simulink model "Template_v3_03_2020a"  (R2020a)
settings: Solver=ode4  StartTime=0.0  StopTime=tsim  FixedStep=baseRate  RelTol=1e-3  EnableMultiTasking=on
values from neighbouring files (symbols this model uses):
  baseRate = 0.05    [Run_Initializer.m]
  dockDist = 0.5    [Run_Initializer.m]
  drop_states_BLACK = [ 1.19; 1.45; -0.06737]    [Run_Initializer.m]
  drop_states_BLUE = [ 0.52; 1.45; -0.06737]    [Run_Initializer.m]
  drop_states_RED = [ 2.114; 1.46; -3.113]    [Run_Initializer.m]
  F_thrusters_BLACK = 0.25.*ones(8,1)    [Run_Initializer.m]
  F_thrusters_BLUE = 0.25.*ones(8,1)    [Run_Initializer.m]
  F_thrusters_RED = 0.25.*ones(8,1)    [Run_Initializer.m]
  final_states_BLACK = [1; 0.5; (0/180*pi)]    [Run_Initializer.m]
  fixed_att = init_states_RED(3)    [Run_Initializer.m]
  guess = [8.968203153403679e+02,-2.543974115068790e+03,0.235869606391541,0.474952865321742,0.474987768379695,0.520000000000000,0.485664087948638,0,0,.1,.1,.1,.1,.1,.1,.1,.1,.1,.1,.1,.1,.1,.1,.1,.1,.1,.2]    [Run_Initializer.m]
  home_states_BLACK = [ xLength/2; yLength/2; 0]    [Run_Initializer.m]
  home_states_BLUE = [ xLength/2-0.4; yLength/2; 0]    [Run_Initializer.m]
  home_states_RED = [ xLength/2+0.4; yLength/2; pi]    [Run_Initializer.m]
  init_states_BLACK = [0.5; 0.5; (0/180*pi)]    [Run_Initializer.m]
  init_states_BLUE = [ xLength/2-0.7; yLength/2; 0]    [Run_Initializer.m]
  init_states_RED = [ 3; 2; 0]    [Run_Initializer.m]
  Kd_tb = 0.4    [Run_Initializer.m]
  Kd_tblue = 0.4    [Run_Initializer.m]
  Kd_tr = 0.4    [Run_Initializer.m]
  Kd_xb = 5    [Run_Initializer.m]
  Kd_xblue = 5    [Run_Initializer.m]
  Kd_xr = 5    [Run_Initializer.m]
  Kd_yb = 5    [Run_Initializer.m]
  Kd_yblue = 5    [Run_Initializer.m]
  Kd_yr = 5    [Run_Initializer.m]
  Kp_tb = 0.1    [Run_Initializer.m]
  Kp_tblue = 0.1    [Run_Initializer.m]
  Kp_tr = 0.1    [Run_Initializer.m]
  Kp_xb = 2    [Run_Initializer.m]
  Kp_xblue = 2    [Run_Initializer.m]
  Kp_xr = 2    [Run_Initializer.m]
  Kp_yb = 2    [Run_Initializer.m]
  Kp_yblue = 2    [Run_Initializer.m]
  Kp_yr = 2    [Run_Initializer.m]
  max_force = F_thrusters_RED(1)*2 * 0.95    [Run_Initializer.m]
  max_torque = 0.13*4    (= 0.52)    [Run_Initializer.m]
  moving_BLACK = [(final_states_BLACK(1)-init_states_BLACK(1))/Phase3_SubPhase2_Duration,(final_states_BLACK(2)-init_states_BLACK(2))/Phase3_SubPhase2_Duration,0]    [Run_Initializer.m]
  noise_variance_BLACK = 0    [Run_Initializer.m]
  noise_variance_BLUE = 0    [Run_Initializer.m]
  noise_variance_RED = 0    [Run_Initializer.m]
  Phase0_End = Phase0_Duration    (= 10)    [Run_Initializer.m]
  Phase1_End = Phase0_Duration + Phase1_Duration    (= 15)    [Run_Initializer.m]
  Phase2_End = Phase0_Duration + Phase1_Duration +                                   Phase2_Duration    (= 35)    [Run_Initializer.m]
  Phase3_Duration = 85    [Run_Initializer.m]
  Phase3_End = Phase0_Duration + Phase1_Duration +                                   Phase2_Duration + Phase3_Duration    (= 120)    [Run_Initializer.m]
  Phase3_SubPhase1_End = Phase2_End + Phase3_SubPhase1_Duration    (= 40)    [Run_Initializer.m]
  Phase3_SubPhase2_Duration = 70    [Run_Initializer.m]
  Phase3_SubPhase2_End = Phase2_End + Phase3_SubPhase1_Duration +                                   Phase3_SubPhase2_Duration    (= 110)    [Run_Initializer.m]
  Phase3_SubPhase3_End = Phase2_End + Phase3_SubPhase1_Duration +                                   Phase3_SubPhase2_Duration +                                  Phase3_SubPhase3_Duration    (= 120)    [Run_Initializer.m]
  Phase3_SubPhase4_End = Phase2_End + Phase3_SubPhase1_Duration +                                   Phase3_SubPhase2_Duration +                                  Phase3_SubPhase3_Duration +                                  Phase3_SubPhase4_Duration    [Run_Initializer.m]
  Phase4_End = Phase0_Duration + Phase1_Duration +                                   Phase2_Duration + Phase3_Duration +                                   Phase4_Duration    (= 140)    [Run_Initializer.m]
  Phase5_End = Phase0_Duration + Phase1_Duration +                                   Phase2_Duration + Phase3_Duration +                                   Phase4_Duration + Phase5_Duration    (= 145)    [Run_Initializer.m]
  REDInertia = 0.2709    [Run_Initializer.m]
  REDMass = 16.9478    [Run_Initializer.m]
  serverRate = 0.1    [Run_Initializer.m]
  thruster_dist2CG_BLACK = [83.42;-52.58;55.94;-60.05;54.08;-53.92;77.06;-55.94]    [Run_Initializer.m]
  thruster_dist2CG_BLUE = [83.42;-52.58;55.94;-60.05;54.08;-53.92;77.06;-55.94]    [Run_Initializer.m]
  thruster_dist2CG_RED = [49.92;-78.08;70.46;-63.54;81.08;-50.42;57.44;-75.96]    [Run_Initializer.m]
  tolSGRA = [Er; Eg]    [Run_Initializer.m]
  xLength = 3.51155    [Run_Initializer.m]
  yLength = 2.41935    [Run_Initializer.m]
undefined symbols (not defined in the file or in its folder): DiscIntNeverNeededParam, platformSelection, simMode, WhoAmI
libraries: embdlinuxlib x11, raspberrypiBasiclib x10, dspsigops x3, dspswit3 x2, MainLibrary x2, simulink x1
(part 2 of 9)

== system Template_v3_03_2020a/Real-Time Visualization ==
  Set Universal Time (If this is a simulation) : Clock
  UDP Send : embdlinuxlib/UDP Send  remoteURL='172.24.1.102'  remotePort=26000  localURL='0.0.0.0'  localPortSource=Automatically determine  localPort=-1  sampletime=-1  blockPlatform=Raspberry Pi  separateLengthPort=0
      settings: SourceProductBaseCode=SC_BEAGLEBONE_BLUE,RASPPI
  wires:
  Set Universal Time (If this is a simulation)/1 -> UDP Send/1

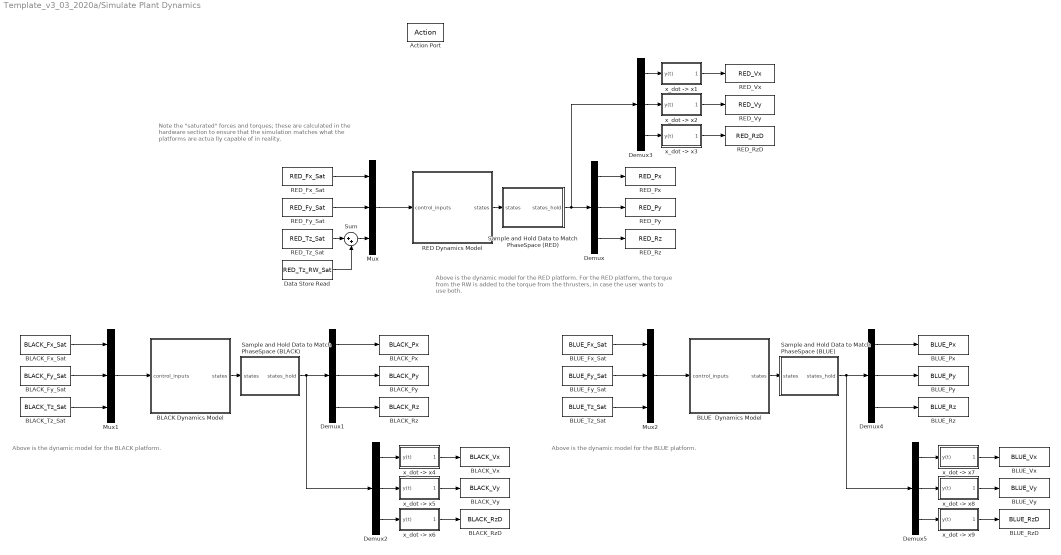
== system Template_v3_03_2020a/Simulate Plant Dynamics ==
  note: Above is the dynamic model for the RED
      | platform. For the RED platform, the torque from the RW is added to the torque from the thrusters, in case the user wants to use both.
  note: Above is the dynamic model for the BLACK platform.
  note: Note the "saturated" forces and torques; these are calculated in the hardware section to ensure that the simulation matches what the platforms are actua lly capable of in reality.
  note: Above is the dynamic model for the BLUE platform.
  Action Port : ActionPort  ActionPortLabel=if(u1 == 1)
  BLACK Dynamics Model : Subsystem  SystemSampleTime=serverRate
  BLACK_Fx_Sat : DataStoreRead  DataStoreName=BLACK_Fx_Sat
  BLACK_Fy_Sat : DataStoreRead  DataStoreName=BLACK_Fy_Sat
  BLACK_Px : DataStoreWrite  DataStoreName=BLACK_Px
  BLACK_Py : DataStoreWrite  DataStoreName=BLACK_Py
  BLACK_Rz : DataStoreWrite  DataStoreName=BLACK_Rz
  BLACK_RzD : DataStoreWrite  DataStoreName=BLACK_RzD
  BLACK_Tz_Sat : DataStoreRead  DataStoreName=BLACK_Tz_Sat
  BLACK_Vx : DataStoreWrite  DataStoreName=BLACK_Vx
  BLACK_Vy : DataStoreWrite  DataStoreName=BLACK_Vy
  BLUE  Dynamics Model : Subsystem  SystemSampleTime=serverRate
  "BLUE_Fx_Sat " : DataStoreRead  DataStoreName=BLUE_Fx_Sat
  BLUE_Fy_Sat : DataStoreRead  DataStoreName=BLUE_Fy_Sat
  "BLUE_Px " : DataStoreWrite  DataStoreName=BLUE_Px
  BLUE_Py : DataStoreWrite  DataStoreName=BLUE_Py
  BLUE_Rz : DataStoreWrite  DataStoreName=BLUE_Rz
  BLUE_RzD : DataStoreWrite  DataStoreName=BLUE_RzD
  BLUE_Tz_Sat : DataStoreRead  DataStoreName=BLUE_Tz_Sat
  BLUE_Vx : DataStoreWrite  DataStoreName=BLUE_Vx
  BLUE_Vy : DataStoreWrite  DataStoreName=BLUE_Vy
  Data Store Read : DataStoreRead  DataStoreName=RED_Tz_RW_Sat
  Demux{,1..5} (6 alike) : Demux  Outputs=3
  Mux : Mux  Inputs=3
  Mux1 : Mux  Inputs=3
  Mux2 : Mux  Inputs=3
  RED Dynamics Model : Subsystem  SystemSampleTime=serverRate
  RED_Fx_Sat : DataStoreRead  DataStoreName=RED_Fx_Sat
  RED_Fy_Sat : DataStoreRead  DataStoreName=RED_Fy_Sat
  RED_Px : DataStoreWrite  DataStoreName=RED_Px
  RED_Py : DataStoreWrite  DataStoreName=RED_Py
  RED_Rz : DataStoreWrite  DataStoreName=RED_Rz
  RED_RzD : DataStoreWrite  DataStoreName=RED_RzD
  RED_Tz_Sat : DataStoreRead  DataStoreName=RED_Tz_Sat
  RED_Vx : DataStoreWrite  DataStoreName=RED_Vx
  RED_Vy : DataStoreWrite  DataStoreName=RED_Vy
  Sample and Hold Data to Match PhaseSpace (BLACK) : Subsystem
  Sample and Hold Data to Match PhaseSpace (BLUE) : Subsystem
  Sample and Hold Data to Match PhaseSpace (RED) : Subsystem
  Sum : Sum  Inputs=|++
  "x_dot -> x1" : Subsystem
  "x_dot -> x2" : Subsystem
  "x_dot -> x3" : Subsystem
  "x_dot -> x4" : Subsystem
  "x_dot -> x5" : Subsystem
  "x_dot -> x6" : Subsystem
  "x_dot -> x7" : Subsystem
  "x_dot -> x8" : Subsystem
  "x_dot -> x9" : Subsystem
  wires:
  Demux/3 -> RED_Rz/1
  RED_Fx_Sat/1 -> Mux/1
  BLACK_Fy_Sat/1 -> Mux1/2
  BLACK_Tz_Sat/1 -> Mux1/3
  RED_Fy_Sat/1 -> Mux/2
  BLACK_Fx_Sat/1 -> Mux1/1
  Demux/2 -> RED_Py/1
  Demux/1 -> RED_Px/1
  Demux1/1 -> BLACK_Px/1
  Demux1/2 -> BLACK_Py/1
  Demux1/3 -> BLACK_Rz/1
  RED_Tz_Sat/1 -> Sum/1
  Sum/1 -> Mux/3
  Data Store Read/1 -> Sum/2
  Demux2/1 -> "x_dot -> x4"/1(y(t))
  Demux2/2 -> "x_dot -> x5"/1(y(t))
  Demux2/3 -> "x_dot -> x6"/1(y(t))
  Demux3/2 -> "x_dot -> x2"/1(y(t))
  Demux3/1 -> "x_dot -> x1"/1(y(t))
  Demux3/3 -> "x_dot -> x3"/1(y(t))
  "x_dot -> x1"/1(dy(t)/dt) -> RED_Vx/1
  "x_dot -> x2"/1(dy(t)/dt) -> RED_Vy/1
  "x_dot -> x3"/1(dy(t)/dt) -> RED_RzD/1
  "x_dot -> x4"/1(dy(t)/dt) -> BLACK_Vx/1
  "x_dot -> x5"/1(dy(t)/dt) -> BLACK_Vy/1
  "x_dot -> x6"/1(dy(t)/dt) -> BLACK_RzD/1
  Mux/1 -> RED Dynamics Model/1(control_inputs)
  Mux1/1 -> BLACK Dynamics Model/1(control_inputs)
  Sample and Hold Data to Match PhaseSpace (BLACK)/1(states_hold) -> Demux2/1, Demux1/1
  BLACK Dynamics Model/1(states) -> Sample and Hold Data to Match PhaseSpace (BLACK)/1(states)
  Sample and Hold Data to Match PhaseSpace (RED)/1("states_hold ") -> Demux3/1, Demux/1
  RED Dynamics Model/1(states) -> Sample and Hold Data to Match PhaseSpace (RED)/1(states)
  Demux4/3 -> BLUE_Rz/1
  Demux5/3 -> "x_dot -> x9"/1(y(t))
  Demux4/1 -> "BLUE_Px "/1
  "x_dot -> x9"/1(dy(t)/dt) -> BLUE_RzD/1
  "x_dot -> x8"/1(dy(t)/dt) -> BLUE_Vy/1
  BLUE  Dynamics Model/1(states) -> Sample and Hold Data to Match PhaseSpace (BLUE)/1(states)
  Sample and Hold Data to Match PhaseSpace (BLUE)/1(states_hold) -> Demux5/1, Demux4/1
  "BLUE_Fx_Sat "/1 -> Mux2/1
  BLUE_Fy_Sat/1 -> Mux2/2
  BLUE_Tz_Sat/1 -> Mux2/3
  Mux2/1 -> BLUE  Dynamics Model/1(control_inputs)
  Demux5/1 -> "x_dot -> x7"/1(y(t))
  Demux5/2 -> "x_dot -> x8"/1(y(t))
  "x_dot -> x7"/1(dy(t)/dt) -> BLUE_Vx/1
  Demux4/2 -> BLUE_Py/1

== system Template_v3_03_2020a/Subsystem ==
  Universal_Time : DataStoreRead  DataStoreName=Univ_Time
  Time : Outport  VectorParamsAs1DForOutWhenUnconnected=off
  wires:
  Universal_Time/1 -> Time/1

== system Template_v3_03_2020a/Float & Magnet Controls/Change RED Behavior ==
  Action Port : ActionPort  ActionPortLabel=if(u1 == 0)
  Data Store Read : DataStoreRead  DataStoreName=Magnet_State
  Data Store Read1 : DataStoreRead  DataStoreName=Float_State
  GPIO for Magnet : embdlinuxlib/GPIO Write  board=Pi 3 Model B  gpio=10  direction=Output  blockPlatform=Raspberry Pi
      settings: SourceProductBaseCode=SC_BEAGLEBONE_BLUE,RASPPI
  GPIO for Pucks : embdlinuxlib/GPIO Write  board=Pi 3 Model B  gpio=26  direction=Output  blockPlatform=Raspberry Pi
      settings: SourceProductBaseCode=SC_BEAGLEBONE_BLUE,RASPPI
  wires:
  Data Store Read1/1 -> GPIO for Pucks/1
  Data Store Read/1 -> GPIO for Magnet/1

== system Template_v3_03_2020a/Float & Magnet Controls/Is this a simulation? ==
  Constant : Constant  Value=simMode  SampleTime=-1
  isSim : Outport  VectorParamsAs1DForOutWhenUnconnected=off
  wires:
  Constant/1 -> isSim/1

== system Template_v3_03_2020a/From Force//Torque to PWM Signal/Change BLACK Behavior ==
  note: Calculate the percentage of time each thruster must be on, and send to the PWM blocks.
  note: Using the attitude, rotate the forces into the body frame.
  note: Calculate which thrusters must be turned on and for how long.
  Action Port : ActionPort  ActionPortLabel=if(u1 == 2 | u2 == 1)
  BLACK_Fx : DataStoreRead  DataStoreName=BLACK_Fx
  BLACK_Fy : DataStoreRead  DataStoreName=BLACK_Fy
  BLACK_Rz : DataStoreRead  DataStoreName=BLACK_Rz
  BLACK_Tz : DataStoreRead  DataStoreName=BLACK_Tz
  Calculate Thruster ON/OFF : Subsystem
  Mux : Mux  Inputs=2
  Mux1 : Mux  Inputs=2
  Rotate Forces to Body : Subsystem
  BLACK PWM : Outport  VectorParamsAs1DForOutWhenUnconnected=off
  wires:
  Rotate Forces to Body/1(F_b) -> Mux1/1
  BLACK_Fx/1 -> Mux/1
  Calculate Thruster ON/OFF/1(ThrusterPWM) -> BLACK PWM/1
  BLACK_Rz/1 -> Rotate Forces to Body/2(Rz)
  Mux/1 -> Rotate Forces to Body/1("F_I ")
  BLACK_Tz/1 -> Mux1/2
  Mux1/1 -> Calculate Thruster ON/OFF/1("[Fx_b; Fy_b; Tz]")
  BLACK_Fy/1 -> Mux/2

== system Template_v3_03_2020a/From Force//Torque to PWM Signal/Change BLUE Behavior ==
  note: Calculate the percentage of time each thruster must be on, and send to the PWM blocks.
  note: Using the attitude, rotate the forces into the body frame.
  note: Calculate which thrusters must be turned on and for how long.
  Action Port : ActionPort  ActionPortLabel=if(u1 == 3 | u2 == 1)
  BLUE_Fx : DataStoreRead  DataStoreName=BLUE_Fx
  BLUE_Fy : DataStoreRead  DataStoreName=BLUE_Fy
  BLUE_Rz : DataStoreRead  DataStoreName=BLUE_Rz
  BLUE_Tz : DataStoreRead  DataStoreName=BLUE_Tz
  Calculate Thruster ON/OFF : Subsystem
  Mux : Mux  Inputs=2
  Mux1 : Mux  Inputs=2
  Rotate Forces to Body : Subsystem
  BLUE PWM : Outport  VectorParamsAs1DForOutWhenUnconnected=off
  wires:
  Rotate Forces to Body/1(F_b) -> Mux1/1
  BLUE_Fx/1 -> Mux/1
  Calculate Thruster ON/OFF/1(ThrusterPWM) -> BLUE PWM/1
  BLUE_Rz/1 -> Rotate Forces to Body/2(Rz)
  Mux/1 -> Rotate Forces to Body/1("F_I ")
  BLUE_Tz/1 -> Mux1/2
  Mux1/1 -> Calculate Thruster ON/OFF/1("[Fx_b; Fy_b; Tz]")
  BLUE_Fy/1 -> Mux/2

== system Template_v3_03_2020a/From Force//Torque to PWM Signal/Change RED Behavior ==
  note: Calculate which thrusters must be turned on and for how long.
  note: Using the attitude, rotate the forces into the body frame.
  note: Calculate the percentage of time each thruster must be on, and send to the PWM blocks.
  Action Port : ActionPort  ActionPortLabel=if(u1 == 1 | u2 == 1)
  Calculate Thruster ON/OFF : Subsystem
  Mux : Mux  Inputs=2
  Mux1 : Mux  Inputs=2
  RED_Fx : DataStoreRead  DataStoreName=RED_Fx
  RED_Fy : DataStoreRead  DataStoreName=RED_Fy
  RED_Rz : DataStoreRead  DataStoreName=RED_Rz
  RED_Tz : DataStoreRead  DataStoreName=RED_Tz
  Rotate Forces to Body : Subsystem
  RED PWM : Outport  VectorParamsAs1DForOutWhenUnconnected=off
  wires:
  RED_Tz/1 -> Mux1/2
  Mux/1 -> Rotate Forces to Body/1("F_I ")
  RED_Fy/1 -> Mux/2
  Mux1/1 -> Calculate Thruster ON/OFF/1("[Fx_b; Fy_b; Tz]")
  RED_Fx/1 -> Mux/1
  RED_Rz/1 -> Rotate Forces to Body/2(Rz)
  Rotate Forces to Body/1(F_b) -> Mux1/1
  Calculate Thruster ON/OFF/1(ThrusterPWM) -> RED PWM/1

== system Template_v3_03_2020a/From Force//Torque to PWM Signal/Is this a simulation? ==
  Constant : Constant  Value=simMode  SampleTime=-1
  isSim : Outport  VectorParamsAs1DForOutWhenUnconnected=off
  wires:
  Constant/1 -> isSim/1

== system Template_v3_03_2020a/From Force//Torque to PWM Signal/Send Commands to PWM Blocks ==
  In1 : Inport
  In2 : Inport  Port=2
  In3 : Inport  Port=3
  In4 : Inport  Port=4
  In5 : Inport  Port=5
  In6 : Inport  Port=6
  In7 : Inport  Port=7
  In8 : Inport  Port=8
  In9 : Inport  Port=9
  BLACK T2 : raspberrypiBasiclib/PWM  board=Pi 3 Model B+  Pin_=9  Frequency=10  blockPlatform=Raspberry Pi
      settings: SourceProductBaseCode=RASPPI
  RED T1 - BLACK T8 : raspberrypiBasiclib/PWM  board=Pi 3 Model B+  Pin_=27  Frequency=10  blockPlatform=Raspberry Pi
      settings: SourceProductBaseCode=RASPPI
  RED T2 - BLACK T3 : raspberrypiBasiclib/PWM  board=Pi 3 Model B+  Pin_=19  Frequency=10  blockPlatform=Raspberry Pi
      settings: SourceProductBaseCode=RASPPI
  RED T3 : raspberrypiBasiclib/PWM  board=Pi 3 Model B+  Pin_=4  Frequency=10  blockPlatform=Raspberry Pi
      settings: SourceProductBaseCode=RASPPI
  RED T4 - BLACK T5 : raspberrypiBasiclib/PWM  board=Pi 3 Model B+  Pin_=22  Frequency=10  blockPlatform=Raspberry Pi
      settings: SourceProductBaseCode=RASPPI
  RED T5 - BLACK T4 : raspberrypiBasiclib/PWM  board=Pi 3 Model B+  Pin_=5  Frequency=10  blockPlatform=Raspberry Pi
      settings: SourceProductBaseCode=RASPPI
  RED T6 - BLACK T7 : raspberrypiBasiclib/PWM  board=Pi 3 Model B+  Pin_=6  Frequency=10  blockPlatform=Raspberry Pi
      settings: SourceProductBaseCode=RASPPI
  RED T7 - BLACK T6 : raspberrypiBasiclib/PWM  board=Pi 3 Model B+  Pin_=13  Frequency=10  blockPlatform=Raspberry Pi
      settings: SourceProductBaseCode=RASPPI
  RED T8 - BLACK T1 : raspberrypiBasiclib/PWM  board=Pi 3 Model B+  Pin_=17  Frequency=10  blockPlatform=Raspberry Pi
      settings: SourceProductBaseCode=RASPPI
  wires:
  In4/1 -> RED T4 - BLACK T5/1
  In5/1 -> RED T5 - BLACK T4/1
  In1/1 -> RED T1 - BLACK T8/1
  In8/1 -> RED T8 - BLACK T1/1
  In9/1 -> BLACK T2/1
  In7/1 -> RED T7 - BLACK T6/1
  In6/1 -> RED T6 - BLACK T7/1
  In3/1 -> RED T3/1
  In2/1 -> RED T2 - BLACK T3/1

== system Template_v3_03_2020a/From Torque, Command RW/Change BLACK Behavior ==
  note: BLACK does not currently have the capability to use a RW.
  Action Port : ActionPort  ActionPortLabel=if(u1 == 2 | u2 == 1)

== system Template_v3_03_2020a/From Torque, Command RW/Change BLUE Behavior ==
  note: BLUE does not currently have the capability to use a RW.
  Action Port : ActionPort  ActionPortLabel=if(u1 == 3 | u2 == 1)

== system Template_v3_03_2020a/From Torque, Command RW/Change RED Behavior ==
  note: In this subsection, the commanded torque is converted to an RPM, which is then saturated based on the known limits of the RW
  note: The saturated wheel RPM is then sent to the wheel controller using PWM blocks.
  Action Port : ActionPort  ActionPortLabel=if(u1 == 1 | u2 == 1)
  Calculate Saturated RPM Signal : Subsystem
  RED_Tz_RW : DataStoreRead  DataStoreName=RED_Tz_RW
  RED_Tz_RW_Sat : DataStoreWrite  DataStoreName=RED_Tz_RW_Sat
  Wheel RPM to PWM : Subsystem
  wires:
  Calculate Saturated RPM Signal/2(RPM_Sat) -> RED_Tz_RW_Sat/1
  RED_Tz_RW/1 -> Calculate Saturated RPM Signal/1(Tz)
  Calculate Saturated RPM Signal/1(RPM) -> Wheel RPM to PWM/1(WheelRPM)

== system Template_v3_03_2020a/From Torque, Command RW/Is this a simulation? ==
  Constant : Constant  Value=simMode  SampleTime=-1
  isSim : Outport  VectorParamsAs1DForOutWhenUnconnected=off
  wires:
  Constant/1 -> isSim/1

== system Template_v3_03_2020a/Grab PhaseSpace Data via UDP/Initialize Universal Time (Simulation) ==
  Action Port : ActionPort  ActionPortLabel=elseif(u1 == 1)
  Set Universal Time (If this is a simulation) : Clock
  Universal_Time : DataStoreWrite  DataStoreName=Univ_Time
  wires:
  Set Universal Time (If this is a simulation)/1 -> Universal_Time/1

== system Template_v3_03_2020a/Grab PhaseSpace Data via UDP/Is this a simulation?1 ==
  Constant : Constant  Value=simMode  SampleTime=-1
  isSim : Outport  VectorParamsAs1DForOutWhenUnconnected=off
  wires:
  Constant/1 -> isSim/1

== system Template_v3_03_2020a/Grab PhaseSpace Data via UDP/Use Hardware to Obtain States ==
  note: Because the UDP block binds to the first platofrm that it sees, it is not currently possible to run RED+BLACK without having RED send BLACK the data packets.
  Action Port : ActionPort  ActionPortLabel=if(u1 == 0)
  "Check whether both platforms are being used, and if so then use RED to send data to BLACK " : If  IfExpression=u1 == 1 | u1 == 2 | u1 == 5  ElseIfExpressions=u1 == 3| u1 == 4  ShowElse=off
  "Using RED+BLACK, or RED+BLACK+ARM" : Subsystem  TreatAsAtomicUnit=on
  "Using RED, BLACK, BLUE, or RED + ARM" : Subsystem  TreatAsAtomicUnit=on
  Which PLATFORM is being used? : Constant  Value=platformSelection  SampleTime=-1
  wires:
  "Check whether both platforms are being used, and if so then use RED to send data to BLACK "/1 -> "Using RED, BLACK, BLUE, or RED + ARM"/Action
  "Check whether both platforms are being used, and if so then use RED to send data to BLACK "/2 -> "Using RED+BLACK, or RED+BLACK+ARM"/Action
  Which PLATFORM is being used?/1 -> "Check whether both platforms are being used, and if so then use RED to send data to BLACK "/1

== system Template_v3_03_2020a/Phase #0: Wait for Synchronization/Change BLACK Behavior ==
  note: Before getting good data, the platforms must NOT be floating. So, float is set to be "off".
  note: For the initialization phase, we do not want any thrust. Thus, all commanded forces are zero.
  Action Port : ActionPort  ActionPortLabel=if(u1 == 2 | u2 == 1)
  BLACK_Fx : DataStoreWrite  DataStoreName=BLACK_Fx
  BLACK_Fy : DataStoreWrite  DataStoreName=BLACK_Fy
  BLACK_Tz : DataStoreWrite  DataStoreName=BLACK_Tz
  Constant3 : Constant  Value=0
  Constant4 : Constant  Value=0
  Constant5 : Constant  Value=0
  Data Store Write4 : DataStoreWrite  DataStoreName=Float_State
  Puck State : Constant  Value=0
  wires:
  Constant3/1 -> BLACK_Fx/1
  Constant5/1 -> BLACK_Tz/1
  Constant4/1 -> BLACK_Fy/1
  Puck State/1 -> Data Store Write4/1

== system Template_v3_03_2020a/Phase #0: Wait for Synchronization/Change BLUE Behavior ==
  note: Before getting good data, the platforms must NOT be floating. So, float is set to be "off".
  note: For the initialization phase, we do not want any thrust. Thus, all commanded forces are zero.
  Action Port : ActionPort  ActionPortLabel=if(u1 == 3 | u2 == 1)
  BLUE_Fx : DataStoreWrite  DataStoreName=BLUE_Fx
  BLUE_Fy : DataStoreWrite  DataStoreName=BLUE_Fy
  BLUE_Tz : DataStoreWrite  DataStoreName=BLUE_Tz
  Constant3 : Constant  Value=0
  Constant4 : Constant  Value=0
  Constant5 : Constant  Value=0
  Data Store Write4 : DataStoreWrite  DataStoreName=Float_State
  Puck State : Constant  Value=0
  wires:
  Constant3/1 -> BLUE_Fx/1
  Constant5/1 -> BLUE_Tz/1
  Constant4/1 -> BLUE_Fy/1
  Puck State/1 -> Data Store Write4/1

== system Template_v3_03_2020a/Phase #0: Wait for Synchronization/Change RED Behavior ==
  note: For the initialization phase, we do not want any thrust or movement from the robotic arm. Thus, all commanded forces are zero.
  note: Before getting good data, the platforms must NOT be floating. So, float is set to be "off".
  Action Port : ActionPort  ActionPortLabel=if(u1 == 1 | u2 == 1)
  Constant{,1..6} (7 alike) : Constant  Value=0
  Data Store Write : DataStoreWrite  DataStoreName=RED_Tz_Shoulder
  Data Store Write1 : DataStoreWrite  DataStoreName=RED_Tz_Elbow
  Data Store Write2 : DataStoreWrite  DataStoreName=RED_Tz_Wrist
  Data Store Write4 : DataStoreWrite  DataStoreName=Float_State
  Puck State : Constant  Value=0
  RED_Fx : DataStoreWrite  DataStoreName=RED_Fx
  RED_Fy : DataStoreWrite  DataStoreName=RED_Fy
  RED_Tz : DataStoreWrite  DataStoreName=RED_Tz
  RED_Tz_RW : DataStoreWrite  DataStoreName=RED_Tz_RW
  wires:
  Constant1/1 -> RED_Fy/1
  Constant2/1 -> RED_Tz/1
  Constant/1 -> RED_Fx/1
  Constant4/1 -> Data Store Write/1
  Constant5/1 -> Data Store Write1/1
  Constant6/1 -> Data Store Write2/1
  Constant3/1 -> RED_Tz_RW/1
  Puck State/1 -> Data Store Write4/1

== system Template_v3_03_2020a/Phase #0: Wait for Synchronization/Is this a simulation? ==
  Constant : Constant  Value=simMode  SampleTime=-1
  isSim : Outport  VectorParamsAs1DForOutWhenUnconnected=off
  wires:
  Constant/1 -> isSim/1

== system Template_v3_03_2020a/Phase #1: Start Floating /Change BLACK Behavior ==
  note: For the float phase, we do not want any thrust. Thus, all commanded forces are zero.
  note: Now that good data is available, the platform can start to float.
  Action Port : ActionPort  ActionPortLabel=if(u1 == 2 | u2 == 1)
  BLACK_Fx : DataStoreWrite  DataStoreName=BLACK_Fx
  BLACK_Fy : DataStoreWrite  DataStoreName=BLACK_Fy
  BLACK_Tz : DataStoreWrite  DataStoreName=BLACK_Tz
  Constant3 : Constant  Value=0
  Constant4 : Constant  Value=0
  Constant5 : Constant  Value=0
  Data Store Write4 : DataStoreWrite  DataStoreName=Float_State
  Puck State : Constant
  wires:
  Constant3/1 -> BLACK_Fx/1
  Constant5/1 -> BLACK_Tz/1
  Constant4/1 -> BLACK_Fy/1
  Puck State/1 -> Data Store Write4/1

== system Template_v3_03_2020a/Phase #1: Start Floating /Change BLUE Behavior ==
  note: Before getting good data, the platforms must NOT be floating. So, float is set to be "off".
  note: For the initialization phase, we do not want any thrust. Thus, all commanded forces are zero.
  Action Port : ActionPort  ActionPortLabel=if(u1 == 3 | u2 == 1)
  BLUE_Fx : DataStoreWrite  DataStoreName=BLUE_Fx
  BLUE_Fy : DataStoreWrite  DataStoreName=BLUE_Fy
  BLUE_Tz : DataStoreWrite  DataStoreName=BLUE_Tz
  Constant3 : Constant  Value=0
  Constant4 : Constant  Value=0
  Constant5 : Constant  Value=0
  Data Store Write4 : DataStoreWrite  DataStoreName=Float_State
  Puck State : Constant
  wires:
  Constant3/1 -> BLUE_Fx/1
  Constant5/1 -> BLUE_Tz/1
  Constant4/1 -> BLUE_Fy/1
  Puck State/1 -> Data Store Write4/1

== system Template_v3_03_2020a/Phase #1: Start Floating /Change RED Behavior ==
  note: Now that good data is available, the platforms can start to float.
  note: For the float phase, we do not want any thrust or movement from the robotic arm. Thus, all commanded forces are zero.
  Action Port : ActionPort  ActionPortLabel=if(u1 == 1 | u2 == 1)
  Constant{,1..6} (7 alike) : Constant  Value=0
  Data Store Write : DataStoreWrite  DataStoreName=RED_Tz_Shoulder
  Data Store Write1 : DataStoreWrite  DataStoreName=RED_Tz_Elbow
  Data Store Write2 : DataStoreWrite  DataStoreName=RED_Tz_Wrist
  Data Store Write4 : DataStoreWrite  DataStoreName=Float_State
  Puck State : Constant
  RED_Fx : DataStoreWrite  DataStoreName=RED_Fx
  RED_Fy : DataStoreWrite  DataStoreName=RED_Fy
  RED_Tz : DataStoreWrite  DataStoreName=RED_Tz
  RED_Tz_RW : DataStoreWrite  DataStoreName=RED_Tz_RW
  wires:
  Constant/1 -> RED_Fx/1
  Constant3/1 -> RED_Tz_RW/1
  Constant4/1 -> Data Store Write/1
  Constant2/1 -> RED_Tz/1
  Constant6/1 -> Data Store Write2/1
  Constant1/1 -> RED_Fy/1
  Constant5/1 -> Data Store Write1/1
  Puck State/1 -> Data Store Write4/1

== system Template_v3_03_2020a/Phase #1: Start Floating /Is this a simulation? ==
  Constant : Constant  Value=simMode  SampleTime=-1
  isSim : Outport  VectorParamsAs1DForOutWhenUnconnected=off
  wires:
  Constant/1 -> isSim/1

== system Template_v3_03_2020a/Phase #2: Move to Initial Position/Change BLACK Behavior ==
  note: Additional Blocks
  note: PD Control Law - BLACK
  note: Additional blocks are stored here.
  note: A simple PD control law is used here to command the platform to it's initial position, as defined in the initializer.
  Action Port : ActionPort  ActionPortLabel=if(u1 == 2 | u2 == 1)
  BLACK_Fx : DataStoreWrite  DataStoreName=BLACK_Fx
  BLACK_Fy : DataStoreWrite  DataStoreName=BLACK_Fy
  BLACK_Px : DataStoreRead  DataStoreName=BLACK_Px
  "BLACK_Py " : DataStoreRead  DataStoreName=BLACK_Py
  BLACK_Rz : DataStoreRead  DataStoreName=BLACK_Rz
  BLACK_Tz : DataStoreWrite  DataStoreName=BLACK_Tz
  Custom Discrete PD (Attitude) : Subsystem
  Custom Discrete PD (X-Position) : Subsystem
  Custom Discrete PD (Y-Position) : Subsystem
  Data Store Write3 : DataStoreWrite  DataStoreName=Float_State
  Desired Attitude (BLACK) : Constant  Value=init_states_BLACK(3)  SampleTime=-1
  Desired Px (BLACK) : Constant  Value=init_states_BLACK(1)  SampleTime=-1
  Desired Py (BLACK) : Constant  Value=init_states_BLACK(2)  SampleTime=-1
  Hough Control : Subsystem
  Puck State : Constant
  Subtract : Sum  Inputs=+-
  Subtract1 : Sum  Inputs=+-
  wires:
  Custom Discrete PD (Y-Position)/1(Fy) -> BLACK_Fy/1
  Hough Control/1(Err) -> Custom Discrete PD (Attitude)/1(ez)
  BLACK_Px/1 -> Subtract/2
  Subtract1/1 -> Custom Discrete PD (Y-Position)/1(ey)
  Custom Discrete PD (Attitude)/1(Tz) -> BLACK_Tz/1
  "BLACK_Py "/1 -> Subtract1/2
  Subtract/1 -> Custom Discrete PD (X-Position)/1(ex)
  Custom Discrete PD (X-Position)/1(Fx) -> BLACK_Fx/1
  Desired Px (BLACK)/1 -> Subtract/1
  Desired Py (BLACK)/1 -> Subtract1/1
  Desired Attitude (BLACK)/1 -> Hough Control/1(Ref)
  BLACK_Rz/1 -> Hough Control/2(Act)
  Puck State/1 -> Data Store Write3/1

== system Template_v3_03_2020a/Phase #2: Move to Initial Position/Change BLUE Behavior ==
  note: PD Control Law - BLUE
  note: Additional blocks are stored here.
  note: A simple PD control law is used here to command the platform to it's initial position, as defined in the initializer.
  note: Additional Blocks
  Action Port : ActionPort  ActionPortLabel=if(u1 == 3 | u2 == 1)
  BLUE_Fx : DataStoreWrite  DataStoreName=BLUE_Fx
  BLUE_Fy : DataStoreWrite  DataStoreName=BLUE_Fy
  BLUE_Px : DataStoreRead  DataStoreName=BLUE_Px
  "BLUE_Py " : DataStoreRead  DataStoreName=BLUE_Py
  BLUE_Rz : DataStoreRead  DataStoreName=BLUE_Rz
  BLUE_Tz : DataStoreWrite  DataStoreName=BLUE_Tz
  Custom Discrete PD (Attitude) : Subsystem
  Custom Discrete PD (X-Position) : Subsystem
  Custom Discrete PD (Y-Position) : Subsystem
  Data Store Write3 : DataStoreWrite  DataStoreName=Float_State
  Desired Attitude (BLUE) : Constant  Value=init_states_BLUE(3)  SampleTime=-1
  Desired Px (BLUE) : Constant  Value=init_states_BLUE(1)  SampleTime=-1
  Desired Py (BLUE) : Constant  Value=init_states_BLUE(2)  SampleTime=-1
  Hough Control : Subsystem
  Puck State : Constant
  Subtract : Sum  Inputs=+-
  Subtract1 : Sum  Inputs=+-
  wires:
  Desired Attitude (BLUE)/1 -> Hough Control/1(Ref)
  BLUE_Rz/1 -> Hough Control/2(Act)
  Puck State/1 -> Data Store Write3/1
  Subtract/1 -> Custom Discrete PD (X-Position)/1(ex)
  Hough Control/1(Err) -> Custom Discrete PD (Attitude)/1(ez)
  Custom Discrete PD (X-Position)/1(Fx) -> BLUE_Fx/1
  Desired Py (BLUE)/1 -> Subtract1/1
  BLUE_Px/1 -> Subtract/2
  Subtract1/1 -> Custom Discrete PD (Y-Position)/1(ey)
  Desired Px (BLUE)/1 -> Subtract/1
  "BLUE_Py "/1 -> Subtract1/2
  Custom Discrete PD (Y-Position)/1(Fy) -> BLUE_Fy/1
  Custom Discrete PD (Attitude)/1(Tz) -> BLUE_Tz/1

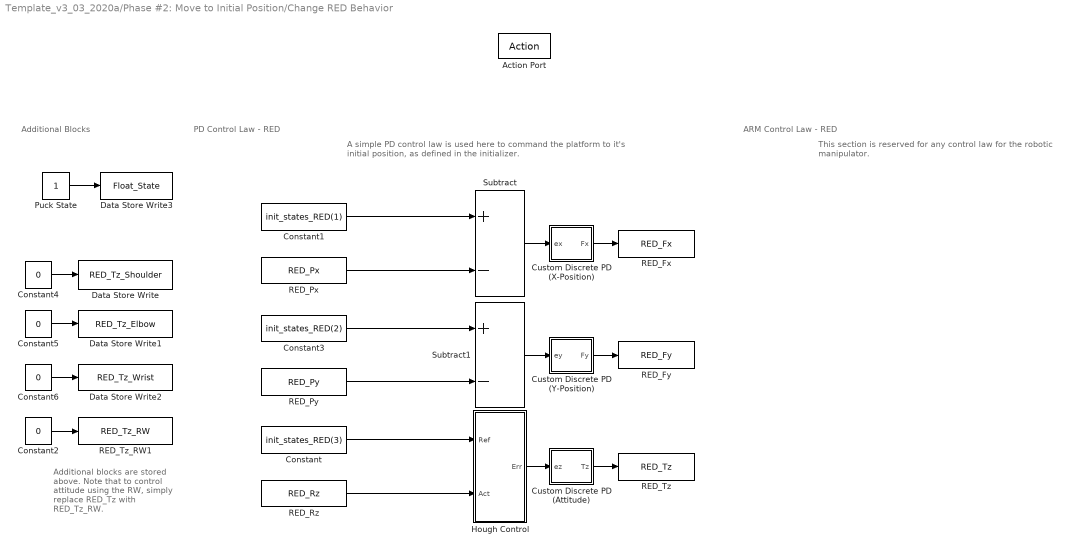
== system Template_v3_03_2020a/Phase #2: Move to Initial Position/Change RED Behavior ==
  note: ARM Control Law - RED
  note: PD Control Law - RED
  note: Additional Blocks
  note: Additional blocks are stored above. Note that to control attitude using the RW, simply replace RED_Tz with RED_Tz_RW.
  note: A simple PD control law is used here to command the platform to it's initial position, as defined in the initializer.
  note: This section is reserved for any control law for the robotic manipulator.
  Action Port : ActionPort  ActionPortLabel=if(u1 == 1 | u2 == 1)
  Constant : Constant  Value=init_states_RED(3)
  Constant1 : Constant  Value=init_states_RED(1)
  Constant{2,4..6} (4 alike) : Constant  Value=0
  Constant3 : Constant  Value=init_states_RED(2)
  Custom Discrete PD (Attitude) : Subsystem
  Custom Discrete PD (X-Position) : Subsystem
  Custom Discrete PD (Y-Position) : Subsystem
  Data Store Write : DataStoreWrite  DataStoreName=RED_Tz_Shoulder
  Data Store Write1 : DataStoreWrite  DataStoreName=RED_Tz_Elbow
  Data Store Write2 : DataStoreWrite  DataStoreName=RED_Tz_Wrist
  Data Store Write3 : DataStoreWrite  DataStoreName=Float_State
  Hough Control : Subsystem
  Puck State : Constant
  RED_Fx : DataStoreWrite  DataStoreName=RED_Fx
  RED_Fy : DataStoreWrite  DataStoreName=RED_Fy
  RED_Px : DataStoreRead  DataStoreName=RED_Px
  "RED_Py " : DataStoreRead  DataStoreName=RED_Py
  RED_Rz : DataStoreRead  DataStoreName=RED_Rz
  RED_Tz : DataStoreWrite  DataStoreName=RED_Tz
  RED_Tz_RW1 : DataStoreWrite  DataStoreName=RED_Tz_RW
  Subtract : Sum  Inputs=+-
  Subtract1 : Sum  Inputs=+-
  wires:
  Constant6/1 -> Data Store Write2/1
  Constant5/1 -> Data Store Write1/1
  Constant2/1 -> RED_Tz_RW1/1
  Constant4/1 -> Data Store Write/1
  Custom Discrete PD (Attitude)/1(Tz) -> RED_Tz/1
  RED_Rz/1 -> Hough Control/2(Act)
  Custom Discrete PD (X-Position)/1(Fx) -> RED_Fx/1
  Subtract/1 -> Custom Discrete PD (X-Position)/1(ex)
  Hough Control/1(Err) -> Custom Discrete PD (Attitude)/1(ez)
  Custom Discrete PD (Y-Position)/1(Fy) -> RED_Fy/1
  RED_Px/1 -> Subtract/2
  "RED_Py "/1 -> Subtract1/2
  Subtract1/1 -> Custom Discrete PD (Y-Position)/1(ey)
  Constant1/1 -> Subtract/1
  Constant3/1 -> Subtract1/1
  Constant/1 -> Hough Control/1(Ref)
  Puck State/1 -> Data Store Write3/1

== system Template_v3_03_2020a/Phase #2: Move to Initial Position/Is this a simulation? ==
  Constant : Constant  Value=simMode  SampleTime=-1
  isSim : Outport  VectorParamsAs1DForOutWhenUnconnected=off
  wires:
  Constant/1 -> isSim/1

== system Template_v3_03_2020a/Phase #3: Experiment/Change BLACK Behavior ==
  note: For experiments, it is usually desirable to have various sub-phases. The sub-phases are defined in the initializer; note that in the template only three sub-phases are present, but more can be added.
  Action Port : ActionPort  ActionPortLabel=if(u1 == 2 | u2 == 1)
  Constant1 : Constant  Value=Phase3_SubPhase2_End  SampleTime=-1
  Constant2 : Constant  Value=Phase3_SubPhase3_End  SampleTime=-1
  Constant3 : Constant  Value=Phase3_SubPhase4_End  SampleTime=-1
  Constant4 : Constant  Value=Phase3_SubPhase1_End  SampleTime=-1
  Experiment Sub-Phases : If  NumInputs=5  IfExpression=u1 < u2  ElseIfExpressions=u1 < u3, u1 < u4, u1 < u5  ShowElse=off
  Sub-Phase #1 : Subsystem  TreatAsAtomicUnit=on
  Sub-Phase #2 1 : Subsystem  TreatAsAtomicUnit=on
  Sub-Phase #3 1 : Subsystem  TreatAsAtomicUnit=on
  Sub-Phase #4 : Subsystem  TreatAsAtomicUnit=on
  Subsystem : Subsystem
  wires:
  Experiment Sub-Phases/2 -> Sub-Phase #2 1/Action
  Experiment Sub-Phases/1 -> Sub-Phase #1/Action
  Experiment Sub-Phases/3 -> Sub-Phase #3 1/Action
  Constant1/1 -> Experiment Sub-Phases/3
  Constant2/1 -> Experiment Sub-Phases/4
  Constant4/1 -> Experiment Sub-Phases/2
  Subsystem/1(Time) -> Experiment Sub-Phases/1
  Constant3/1 -> Experiment Sub-Phases/5
  Experiment Sub-Phases/4 -> Sub-Phase #4/Action

== system Template_v3_03_2020a/Phase #3: Experiment/Change BLUE Behavior ==
  Action Port : ActionPort  ActionPortLabel=if(u1 == 3 | u2 == 1)
  Constant1 : Constant  Value=Phase3_SubPhase2_End  SampleTime=-1
  Constant2 : Constant  Value=Phase3_SubPhase3_End  SampleTime=-1
  Constant3 : Constant  Value=Phase3_SubPhase4_End  SampleTime=-1
  Constant4 : Constant  Value=Phase3_SubPhase1_End  SampleTime=-1
  Experiment Sub-Phases : If  NumInputs=5  IfExpression=u1 < u2  ElseIfExpressions=u1 < u3, u1 < u4, u1 < u5  ShowElse=off
  Sub-Phase #1 : Subsystem  TreatAsAtomicUnit=on
  "Sub-Phase #2 " : Subsystem  TreatAsAtomicUnit=on
  "Sub-Phase #3 " : Subsystem  TreatAsAtomicUnit=on
  Sub-Phase #4 : Subsystem  TreatAsAtomicUnit=on
  Subsystem : Subsystem
  wires:
  Constant3/1 -> Experiment Sub-Phases/5
  Experiment Sub-Phases/4 -> Sub-Phase #4/Action
  Subsystem/1(Time) -> Experiment Sub-Phases/1
  Experiment Sub-Phases/1 -> Sub-Phase #1/Action
  Constant2/1 -> Experiment Sub-Phases/4
  Constant4/1 -> Experiment Sub-Phases/2
  Constant1/1 -> Experiment Sub-Phases/3
  Experiment Sub-Phases/3 -> "Sub-Phase #3 "/Action
  Experiment Sub-Phases/2 -> "Sub-Phase #2 "/Action

== system Template_v3_03_2020a/Phase #3: Experiment/Change RED Behavior ==
  note: For experiments, it is usually desirable to have various sub-phases. The sub-phases are defined in the initializer; note that in the template only three sub-phases are present, but more can be added.
  note: Hold Phase
  note: Manoeuvre Phase
  Action Port : ActionPort  ActionPortLabel=if(u1 == 1 | u2 == 1)
  Constant1 : Constant  Value=Phase3_SubPhase2_End  SampleTime=-1
  Constant2 : Constant  Value=Phase3_SubPhase3_End  SampleTime=-1
  Constant3 : Constant  Value=Phase3_SubPhase4_End  SampleTime=-1
  Constant4 : Constant  Value=Phase3_SubPhase1_End  SampleTime=-1
  Experiment Sub-Phases : If  NumInputs=5  IfExpression=u1 < u2  ElseIfExpressions=u1 < u3, u1 < u4, u1 < u5  ShowElse=off
  Sub-Phase #1 : Subsystem  TreatAsAtomicUnit=on
  "Sub-Phase #2 " : Subsystem  TreatAsAtomicUnit=on
  "Sub-Phase #3 " : Subsystem  TreatAsAtomicUnit=on
  Sub-Phase #4 : Subsystem  TreatAsAtomicUnit=on
  Subsystem : Subsystem
  wires:
  Experiment Sub-Phases/1 -> Sub-Phase #1/Action
  Experiment Sub-Phases/2 -> "Sub-Phase #2 "/Action
  Subsystem/1(Time) -> Experiment Sub-Phases/1
  Experiment Sub-Phases/3 -> "Sub-Phase #3 "/Action
  Constant4/1 -> Experiment Sub-Phases/2
  Constant1/1 -> Experiment Sub-Phases/3
  Constant2/1 -> Experiment Sub-Phases/4
  Constant3/1 -> Experiment Sub-Phases/5
  Experiment Sub-Phases/4 -> Sub-Phase #4/Action
  "Sub-Phase #2 "/1(Px) -> "Sub-Phase #3 "/1(Px)
  "Sub-Phase #2 "/2(Py) -> "Sub-Phase #3 "/2(Py)
  "Sub-Phase #2 "/3(Rz) -> "Sub-Phase #3 "/3(Rz)

== system Template_v3_03_2020a/Phase #3: Experiment/Is this a simulation? ==
  Constant : Constant  Value=simMode  SampleTime=-1
  isSim : Outport  VectorParamsAs1DForOutWhenUnconnected=off
  wires:
  Constant/1 -> isSim/1

== system Template_v3_03_2020a/Phase #4: Return Home/Change BLACK Behavior ==
  note: Additional Blocks
  note: PD Control Law - BLACK
  note: Additional blocks are stored here.
  note: A simple PD control law is used here to command the platform to it's initial position, as defined in the initializer.
  Action Port : ActionPort  ActionPortLabel=if(u1 == 2 | u2 == 1)
  BLACK_Fx : DataStoreWrite  DataStoreName=BLACK_Fx
  BLACK_Fy : DataStoreWrite  DataStoreName=BLACK_Fy
  BLACK_Px : DataStoreRead  DataStoreName=BLACK_Px
  "BLACK_Py " : DataStoreRead  DataStoreName=BLACK_Py
  BLACK_Rz : DataStoreRead  DataStoreName=BLACK_Rz
  BLACK_Tz : DataStoreWrite  DataStoreName=BLACK_Tz
  Custom Discrete PD (Attitude) : Subsystem
  Custom Discrete PD (X-Position) : Subsystem
  Custom Discrete PD (Y-Position) : Subsystem
  Data Store Write3 : DataStoreWrite  DataStoreName=Float_State
  Desired Attitude (BLACK) : Constant  Value=home_states_BLACK(3)  SampleTime=-1
  Desired Px (BLACK) : Constant  Value=home_states_BLACK(1)  SampleTime=-1
  Desired Py (BLACK) : Constant  Value=home_states_BLACK(2)  SampleTime=-1
  Hough Control : Subsystem
  Puck State : Constant
  Subtract : Sum  Inputs=+-
  Subtract1 : Sum  Inputs=+-
  wires:
  Custom Discrete PD (Y-Position)/1(Fy) -> BLACK_Fy/1
  Desired Py (BLACK)/1 -> Subtract1/1
  Hough Control/1(Err) -> Custom Discrete PD (Attitude)/1(ez)
  BLACK_Px/1 -> Subtract/2
  Subtract1/1 -> Custom Discrete PD (Y-Position)/1(ey)
  Custom Discrete PD (Attitude)/1(Tz) -> BLACK_Tz/1
  Desired Attitude (BLACK)/1 -> Hough Control/1(Ref)
  "BLACK_Py "/1 -> Subtract1/2
  Subtract/1 -> Custom Discrete PD (X-Position)/1(ex)
  BLACK_Rz/1 -> Hough Control/2(Act)
  Desired Px (BLACK)/1 -> Subtract/1
  Custom Discrete PD (X-Position)/1(Fx) -> BLACK_Fx/1
  Puck State/1 -> Data Store Write3/1

== system Template_v3_03_2020a/Phase #4: Return Home/Change BLUE Behavior ==
  note: PD Control Law - BLUE
  note: Additional blocks are stored here.
  note: A simple PD control law is used here to command the platform to it's initial position, as defined in the initializer.
  note: Additional Blocks
  Action Port : ActionPort  ActionPortLabel=if(u1 == 3 | u2 == 1)
  BLUE_Fx : DataStoreWrite  DataStoreName=BLUE_Fx
  BLUE_Fy : DataStoreWrite  DataStoreName=BLUE_Fy
  BLUE_Px : DataStoreRead  DataStoreName=BLUE_Px
  "BLUE_Py " : DataStoreRead  DataStoreName=BLUE_Py
  BLUE_Rz : DataStoreRead  DataStoreName=BLUE_Rz
  BLUE_Tz : DataStoreWrite  DataStoreName=BLUE_Tz
  Custom Discrete PD (Attitude) : Subsystem
  Custom Discrete PD (X-Position) : Subsystem
  Custom Discrete PD (Y-Position) : Subsystem
  Data Store Write3 : DataStoreWrite  DataStoreName=Float_State
  Desired Attitude (BLUE) : Constant  Value=home_states_BLUE(3)  SampleTime=-1
  Desired Px (BLUE) : Constant  Value=home_states_BLUE(1)  SampleTime=-1
  Desired Py (BLUE) : Constant  Value=home_states_BLUE(2)  SampleTime=-1
  Hough Control : Subsystem
  Puck State : Constant
  Subtract : Sum  Inputs=+-
  Subtract1 : Sum  Inputs=+-
  wires:
  Puck State/1 -> Data Store Write3/1
  Subtract/1 -> Custom Discrete PD (X-Position)/1(ex)
  Desired Py (BLUE)/1 -> Subtract1/1
  Custom Discrete PD (X-Position)/1(Fx) -> BLUE_Fx/1
  Desired Px (BLUE)/1 -> Subtract/1
  Subtract1/1 -> Custom Discrete PD (Y-Position)/1(ey)
  Hough Control/1(Err) -> Custom Discrete PD (Attitude)/1(ez)
  Desired Attitude (BLUE)/1 -> Hough Control/1(Ref)
  Custom Discrete PD (Attitude)/1(Tz) -> BLUE_Tz/1
  "BLUE_Py "/1 -> Subtract1/2
  Custom Discrete PD (Y-Position)/1(Fy) -> BLUE_Fy/1
  BLUE_Px/1 -> Subtract/2
  BLUE_Rz/1 -> Hough Control/2(Act)

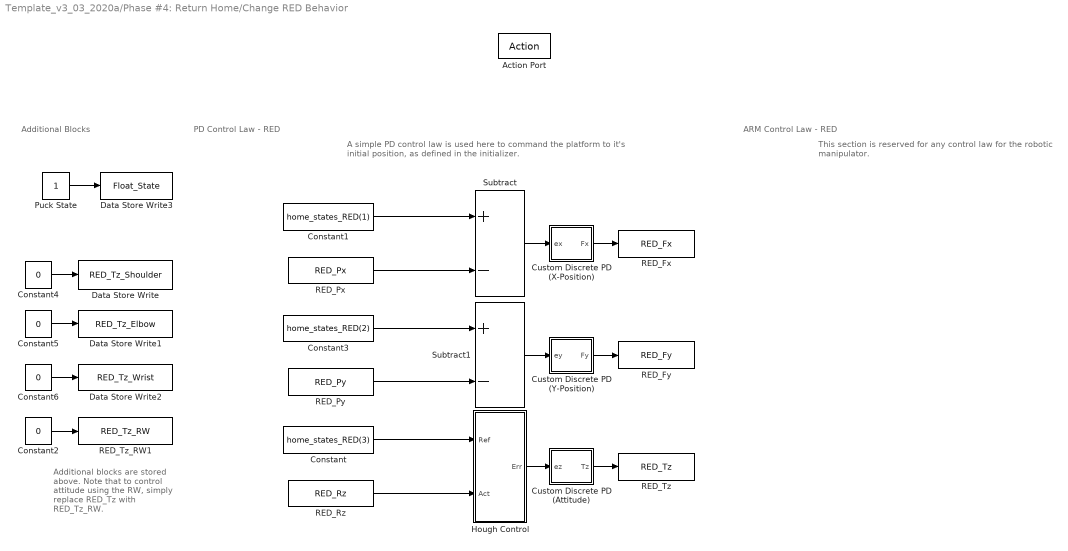
== system Template_v3_03_2020a/Phase #4: Return Home/Change RED Behavior ==
  note: ARM Control Law - RED
  note: PD Control Law - RED
  note: Additional Blocks
  note: Additional blocks are stored above. Note that to control attitude using the RW, simply replace RED_Tz with RED_Tz_RW.
  note: A simple PD control law is used here to command the platform to it's initial position, as defined in the initializer.
  note: This section is reserved for any control law for the robotic manipulator.
  Action Port : ActionPort  ActionPortLabel=if(u1 == 1 | u2 == 1)
  Constant : Constant  Value=home_states_RED(3)
  Constant1 : Constant  Value=home_states_RED(1)
  Constant{2,4..6} (4 alike) : Constant  Value=0
  Constant3 : Constant  Value=home_states_RED(2)
  Custom Discrete PD (Attitude) : Subsystem
  Custom Discrete PD (X-Position) : Subsystem
  Custom Discrete PD (Y-Position) : Subsystem
  Data Store Write : DataStoreWrite  DataStoreName=RED_Tz_Shoulder
  Data Store Write1 : DataStoreWrite  DataStoreName=RED_Tz_Elbow
  Data Store Write2 : DataStoreWrite  DataStoreName=RED_Tz_Wrist
  Data Store Write3 : DataStoreWrite  DataStoreName=Float_State
  Hough Control : Subsystem
  Puck State : Constant
  RED_Fx : DataStoreWrite  DataStoreName=RED_Fx
  RED_Fy : DataStoreWrite  DataStoreName=RED_Fy
  RED_Px : DataStoreRead  DataStoreName=RED_Px
  "RED_Py " : DataStoreRead  DataStoreName=RED_Py
  RED_Rz : DataStoreRead  DataStoreName=RED_Rz
  RED_Tz : DataStoreWrite  DataStoreName=RED_Tz
  RED_Tz_RW1 : DataStoreWrite  DataStoreName=RED_Tz_RW
  Subtract : Sum  Inputs=+-
  Subtract1 : Sum  Inputs=+-
  wires:
  Constant6/1 -> Data Store Write2/1
  Constant5/1 -> Data Store Write1/1
  Constant2/1 -> RED_Tz_RW1/1
  Constant4/1 -> Data Store Write/1
  Constant1/1 -> Subtract/1
  Custom Discrete PD (Attitude)/1(Tz) -> RED_Tz/1
  Constant/1 -> Hough Control/1(Ref)
  RED_Rz/1 -> Hough Control/2(Act)
  Constant3/1 -> Subtract1/1
  Custom Discrete PD (X-Position)/1(Fx) -> RED_Fx/1
  Subtract/1 -> Custom Discrete PD (X-Position)/1(ex)
  Hough Control/1(Err) -> Custom Discrete PD (Attitude)/1(ez)
  Custom Discrete PD (Y-Position)/1(Fy) -> RED_Fy/1
  RED_Px/1 -> Subtract/2
  "RED_Py "/1 -> Subtract1/2
  Subtract1/1 -> Custom Discrete PD (Y-Position)/1(ey)
  Puck State/1 -> Data Store Write3/1

== system Template_v3_03_2020a/Phase #4: Return Home/Is this a simulation? ==
  Constant : Constant  Value=simMode  SampleTime=-1
  isSim : Outport  VectorParamsAs1DForOutWhenUnconnected=off
  wires:
  Constant/1 -> isSim/1

== system Template_v3_03_2020a/Phase #5: Hold Home/Change BLACK Behavior ==
  note: Additional Blocks
  note: PD Control Law - BLACK
  note: A simple PD control law is used here to command the platform to it's initial position, as defined in the initializer.
  note: Additional blocks are stored here.
  Action Port : ActionPort  ActionPortLabel=if(u1 == 2 | u2 == 1)
  BLACK_Fx : DataStoreWrite  DataStoreName=BLACK_Fx
  BLACK_Fy : DataStoreWrite  DataStoreName=BLACK_Fy
  BLACK_Px : DataStoreRead  DataStoreName=BLACK_Px
  "BLACK_Py " : DataStoreRead  DataStoreName=BLACK_Py
  BLACK_Rz : DataStoreRead  DataStoreName=BLACK_Rz
  BLACK_Tz : DataStoreWrite  DataStoreName=BLACK_Tz
  Constant : Constant  Value=home_states_BLACK(1)
  Constant2 : Constant  Value=home_states_BLACK(2)
  Constant3 : Constant  Value=home_states_BLACK(3)
  Custom Discrete PD (Attitude) : Subsystem
  Custom Discrete PD (X-Position) : Subsystem
  Custom Discrete PD (Y-Position) : Subsystem
  Data Store Write3 : DataStoreWrite  DataStoreName=Float_State
  Hough Control : Subsystem
  Puck State : Constant
  Subtract : Sum  Inputs=+-
  Subtract1 : Sum  Inputs=+-
  wires:
  Custom Discrete PD (X-Position)/1(Fx) -> BLACK_Fx/1
  "BLACK_Py "/1 -> Subtract1/2
  Subtract1/1 -> Custom Discrete PD (Y-Position)/1(ey)
  Custom Discrete PD (Y-Position)/1(Fy) -> BLACK_Fy/1
  Constant3/1 -> Hough Control/1(Ref)
  Constant/1 -> Subtract/1
  Constant2/1 -> Subtract1/1
  Subtract/1 -> Custom Discrete PD (X-Position)/1(ex)
  Hough Control/1(Err) -> Custom Discrete PD (Attitude)/1(ez)
  Custom Discrete PD (Attitude)/1(Tz) -> BLACK_Tz/1
  BLACK_Px/1 -> Subtract/2
  BLACK_Rz/1 -> Hough Control/2(Act)
  Puck State/1 -> Data Store Write3/1

== system Template_v3_03_2020a/Phase #5: Hold Home/Change BLUE Behavior ==
  note: PD Control Law - WHITE
  note: Additional blocks are stored here.
  note: A simple PD control law is used here to command the platform to it's initial position, as defined in the initializer.
  note: Additional Blocks
  Action Port : ActionPort  ActionPortLabel=if(u1 == 3 | u2 == 1)
  BLUE_Fx : DataStoreWrite  DataStoreName=BLUE_Fx
  BLUE_Fy : DataStoreWrite  DataStoreName=BLUE_Fy
  BLUE_Px : DataStoreRead  DataStoreName=BLUE_Px
  "BLUE_Py " : DataStoreRead  DataStoreName=BLUE_Py
  BLUE_Rz : DataStoreRead  DataStoreName=BLUE_Rz
  BLUE_Tz : DataStoreWrite  DataStoreName=BLUE_Tz
  Custom Discrete PD (Attitude) : Subsystem
  Custom Discrete PD (X-Position) : Subsystem
  Custom Discrete PD (Y-Position) : Subsystem
  Data Store Write3 : DataStoreWrite  DataStoreName=Float_State
  Desired Attitude (BLUE) : Constant  Value=home_states_BLUE(3)  SampleTime=-1
  Desired Px (BLUE) : Constant  Value=home_states_BLUE(1)  SampleTime=-1
  Desired Py (BLUE) : Constant  Value=home_states_BLUE(2)  SampleTime=-1
  Hough Control : Subsystem
  Puck State : Constant
  Subtract : Sum  Inputs=+-
  Subtract1 : Sum  Inputs=+-
  wires:
  Puck State/1 -> Data Store Write3/1
  Custom Discrete PD (Y-Position)/1(Fy) -> BLUE_Fy/1
  Custom Discrete PD (X-Position)/1(Fx) -> BLUE_Fx/1
  Subtract1/1 -> Custom Discrete PD (Y-Position)/1(ey)
  "BLUE_Py "/1 -> Subtract1/2
  Desired Px (BLUE)/1 -> Subtract/1
  Hough Control/1(Err) -> Custom Discrete PD (Attitude)/1(ez)
  Subtract/1 -> Custom Discrete PD (X-Position)/1(ex)
  Custom Discrete PD (Attitude)/1(Tz) -> BLUE_Tz/1
  BLUE_Rz/1 -> Hough Control/2(Act)
  Desired Py (BLUE)/1 -> Subtract1/1
  BLUE_Px/1 -> Subtract/2
  Desired Attitude (BLUE)/1 -> Hough Control/1(Ref)

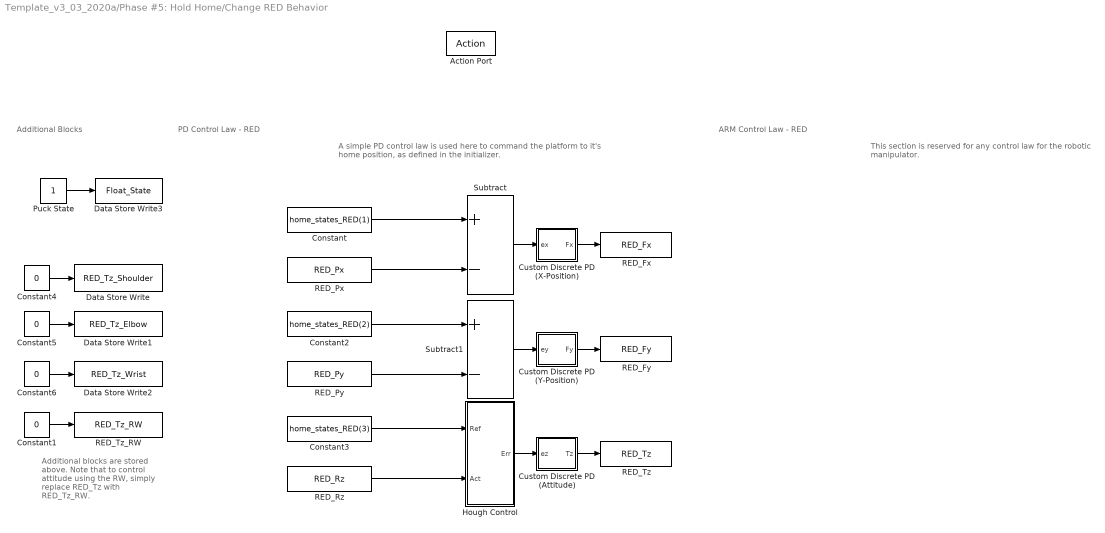
== system Template_v3_03_2020a/Phase #5: Hold Home/Change RED Behavior ==
  note: PD Control Law - RED
  note: ARM Control Law - RED
  note: Additional Blocks
  note: Additional blocks are stored above. Note that to control attitude using the RW, simply replace RED_Tz with RED_Tz_RW.
  note: A simple PD control law is used here to command the platform to it's home position, as defined in the initializer.
  note: This section is reserved for any control law for the robotic manipulator.
  Action Port : ActionPort  ActionPortLabel=if(u1 == 1 | u2 == 1)
  Constant : Constant  Value=home_states_RED(1)
  Constant{1,4..6} (4 alike) : Constant  Value=0
  Constant2 : Constant  Value=home_states_RED(2)
  Constant3 : Constant  Value=home_states_RED(3)
  Custom Discrete PD (Attitude) : Subsystem
  Custom Discrete PD (X-Position) : Subsystem
  Custom Discrete PD (Y-Position) : Subsystem
  Data Store Write : DataStoreWrite  DataStoreName=RED_Tz_Shoulder
  Data Store Write1 : DataStoreWrite  DataStoreName=RED_Tz_Elbow
  Data Store Write2 : DataStoreWrite  DataStoreName=RED_Tz_Wrist
  Data Store Write3 : DataStoreWrite  DataStoreName=Float_State
  Hough Control : Subsystem
  Puck State : Constant
  RED_Fx : DataStoreWrite  DataStoreName=RED_Fx
  RED_Fy : DataStoreWrite  DataStoreName=RED_Fy
  RED_Px : DataStoreRead  DataStoreName=RED_Px
  "RED_Py " : DataStoreRead  DataStoreName=RED_Py
  RED_Rz : DataStoreRead  DataStoreName=RED_Rz
  RED_Tz : DataStoreWrite  DataStoreName=RED_Tz
  RED_Tz_RW : DataStoreWrite  DataStoreName=RED_Tz_RW
  Subtract : Sum  Inputs=+-
  Subtract1 : Sum  Inputs=+-
  wires:
  Constant1/1 -> RED_Tz_RW/1
  Constant5/1 -> Data Store Write1/1
  Constant4/1 -> Data Store Write/1
  Constant6/1 -> Data Store Write2/1
  "RED_Py "/1 -> Subtract1/2
  Custom Discrete PD (Attitude)/1(Tz) -> RED_Tz/1
  Subtract1/1 -> Custom Discrete PD (Y-Position)/1(ey)
  Hough Control/1(Err) -> Custom Discrete PD (Attitude)/1(ez)
  RED_Px/1 -> Subtract/2
  Custom Discrete PD (X-Position)/1(Fx) -> RED_Fx/1
  Subtract/1 -> Custom Discrete PD (X-Position)/1(ex)
  Custom Discrete PD (Y-Position)/1(Fy) -> RED_Fy/1
  Constant/1 -> Subtract/1
  Constant3/1 -> Hough Control/1(Ref)
  RED_Rz/1 -> Hough Control/2(Act)
  Constant2/1 -> Subtract1/1
  Puck State/1 -> Data Store Write3/1

== system Template_v3_03_2020a/Phase #5: Hold Home/Is this a simulation? ==
  Constant : Constant  Value=simMode  SampleTime=-1
  isSim : Outport  VectorParamsAs1DForOutWhenUnconnected=off
  wires:
  Constant/1 -> isSim/1

== system Template_v3_03_2020a/Phase #6: Stop Floating and Spin Down RW/Change BLACK Behavior ==
  note: At the end of the experiment, the pucks must be turned off.
  note: At the end of the experiment, all thrust and arms movement must cease.
  Action Port : ActionPort  ActionPortLabel=if(u1 == 2 | u2 == 1)
  BLACK_Fx : DataStoreWrite  DataStoreName=BLACK_Fx
  BLACK_Fy : DataStoreWrite  DataStoreName=BLACK_Fy
  BLACK_Tz : DataStoreWrite  DataStoreName=BLACK_Tz
  Constant3 : Constant  Value=0
  Constant4 : Constant  Value=0
  Constant5 : Constant  Value=0
  Data Store Write3 : DataStoreWrite  DataStoreName=Float_State
  Puck State : Constant  Value=0
  wires:
  Constant3/1 -> BLACK_Fx/1
  Constant5/1 -> BLACK_Tz/1
  Constant4/1 -> BLACK_Fy/1
  Puck State/1 -> Data Store Write3/1
